simulink model "encoder_test"  (R2022b)
settings: Solver=FixedStepDiscrete  StartTime=0.0  StopTime=10.0  FixedStep=0.01  RelTol=1e-3  EnableMultiTasking=on
libraries: legoev3lib x4
settings Model: ExtModeTrigDuration=2  Creator=hp  LastModifiedBy=hp
settings SolverCC: PositivePriorityOrder=on
settings OptimizationCC: EnhancedBackFolding=on  PassReuseOutputArgsAs=Individual arguments  ZeroExternalMemoryAtStartup=off  ZeroInternalMemoryAtStartup=off  MaxStackSize=64  OptimizeBlockOrder=speed  DifferentSizesBufferReuse=on  OptimizationCustomize=off  EfficientTunableParamExpr=on
settings DebuggingCC: ParameterTunabilityLossMsg=error
settings HardwareCC: ProdBitPerPointer=32  ProdBitPerSizeT=32  ProdBitPerPtrDiffT=32  ProdLargestAtomicInteger=Long  ProdWordSize=32  ProdHWDeviceType=ARM Compatible->ARM 9
settings SFSimCC: MATLABDynamicMemAlloc=off
settings RTWCC: Description=Embedded Coder  SystemTargetFile=ert.tlc  HardwareBoard=LEGO MINDSTORMS EV3  TLCOptions="-aInlineSetEventsForThisBaseRateFcn=TLC_FALSE -aSuppressMultiTaskScheduler=TLC_FALSE  -aRateBasedStepFcn=0"  TemplateMakefile=ert_default_tmf  Toolchain=Sourcery G++ Lite v2009q3
settings CodeAppCC: ForceParamTrailComments=on  IgnoreCustomStorageClasses=off  OperatorAnnotations=on  SimulinkDataObjDesc=on  SFDataObjDesc=on  InsertBlockDesc=on
settings ERTTargetCC: SupportContinuousTime=on  SupportVariableSizeSignals=on  ExtModeTransport=2  ExtModeStaticAlloc=on  ExtModeMexFile=ext_xcp  ExtModeIntrfLevel=Level2 - Open

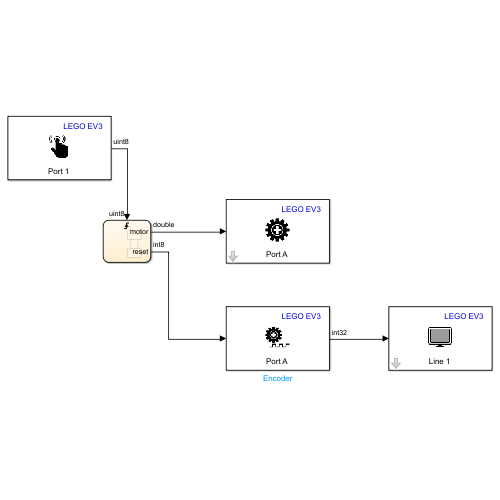
[thumbnail: Simulink's stored preview of the top-level diagram]
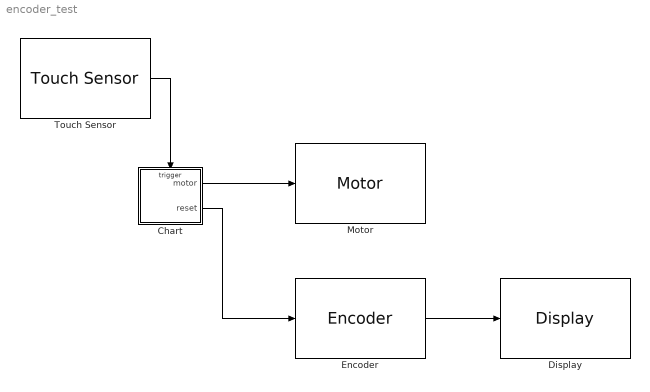
== system encoder_test ==
  Chart : Stateflow chart  TreatAsAtomicUnit=on
  Display : legoev3lib/Display  slcdStr=Angle  slcdLine=1  slcdFormat=Decimal
  Encoder : legoev3lib/Encoder  portNumber=A  opMode=Reset by external signal  sampleTime=0.1
  Motor : legoev3lib/Motor  sportNumber=A  sstopAction=Brake
  Touch Sensor : legoev3lib/Touch Sensor  portNumber=1  sampleTime=0.1
  wires:
  Encoder/1 -> Display/1
  Chart/1(motor) -> Motor/1
  Chart/2(reset) -> Encoder/1
  Touch Sensor/1 -> Chart/Trigger

== stateflow chart encoder_test/Chart ==
  state entry_
    motor = 0;
    reset  = 0;
  state encoder_
    entry:
    motor = 30;
  (default) -> entry_
  encoder_ -> entry_ : buton{reset = 1;}
  entry_ -> encoder_ : buton
  data: motor output; reset output int8
  events: buton input RISING_EDGE_EVENT
